simulink model "SimplerFFTV2"  (R2021b)
settings: Solver=VariableStepAuto  StartTime=0.0  StopTime=3*900/fs  RelTol=1e-3
InitFcn:
  | f = 1000;
  | fs = 18*f;
  | N = 10*fs/f;
  | n = 0:N-1;
  | Ts = 1/fs;
  | t = n*Ts
  | y_n = sin(2*pi*f*n*Ts);
  | Hann = 0.5 * (1 - cos(2*pi*(n/N)))
  | Hamming = 0.54 - 0.46*cos(2*pi*n/N)
undefined symbols (not defined in the file): y_n_Hamming_1Period
libraries: hdlBasic x12, vmcUtilities x1
settings Model: Creator=yxb20126  LastModifiedBy=yxb20126

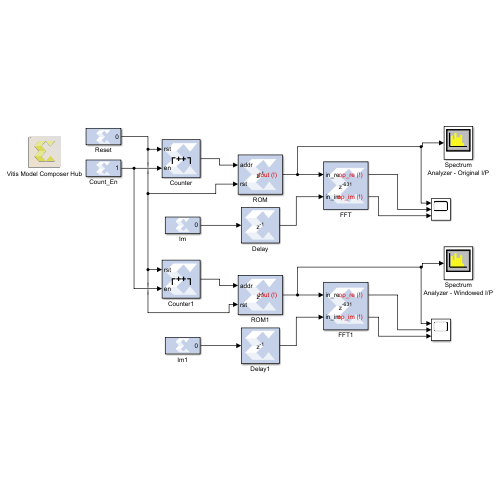
[thumbnail: Simulink's stored preview of the top-level diagram]
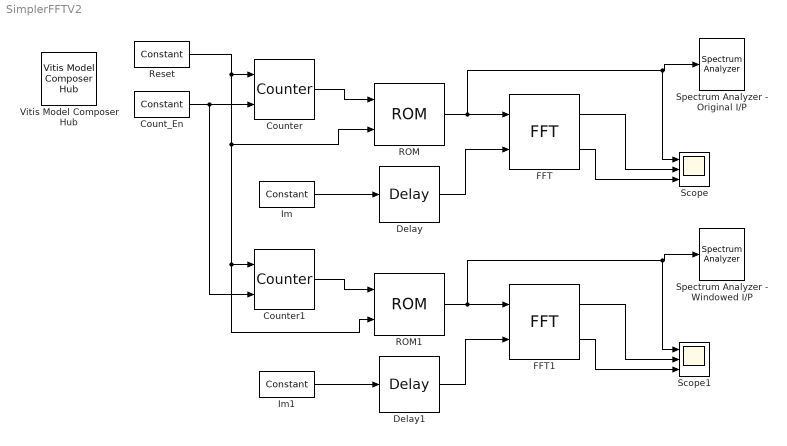
== system SimplerFFTV2 ==
  Count_En : hdlBasic/Constant  const=1  gui_display_data_type=Boolean  arith_type=Boolean  n_bits=16  bin_pt=14  preci_type=Single  exp_width=8  frac_width=24  explicit_period=on  period=1/fs  XmcBlockStatus=1  maskContainerNames=tabcontainer1  block_type=constant  block_config=sysgen:Constant_config
  Counter : hdlBasic/Counter  cnt_type=Count limited  cnt_to=length(y_n)-1  operation=Up  start_count=0  cnt_by_val=1  arith_type=Unsigned  n_bits=8  bin_pt=0  load_pin=off  rst=on  en=on  explicit_period=Explicit  period=1/fs  use_behavioral_HDL=off  implementation=Fabric  XmcBlockStatus=1  maskContainerNames=group1  block_type=counter  block_config=sysgen:Counter_config
  Counter1 : hdlBasic/Counter  cnt_type=Count limited  cnt_to=length(y_n_Hamming_1Period)-1  operation=Up  start_count=0  cnt_by_val=1  arith_type=Unsigned  n_bits=10  bin_pt=0  load_pin=off  rst=on  en=on  explicit_period=Explicit  period=1/fs  use_behavioral_HDL=off  implementation=Fabric  XmcBlockStatus=1  maskContainerNames=group1  block_type=counter  block_config=sysgen:Counter_config
  Delay : hdlBasic/Delay  rst=off  en=off  latency=1  reg_retiming=off  XmcBlockStatus=1  maskContainerNames=group1  block_type=delay  block_config=sysgen:Delay_config
  Delay1 : hdlBasic/Delay  rst=off  en=off  latency=1  reg_retiming=off  XmcBlockStatus=1  maskContainerNames=group1  block_type=delay  block_config=sysgen:Delay_config
  FFT : hdlBasic/FFT  transform_length=512  scale_result_by_fft_length=off  bit_reversed_order=off  optimizegoal=Performance  start_frame=off  simulation_type=fast_sim  simulation_model=sysgen:ForwardFFT_Macro  latency=1  XmcBlockStatus=1  maskContainerNames=group1  block_type=xfft_forward  block_config=sysgen:FFTMacro_config
  FFT1 : hdlBasic/FFT  transform_length=512  scale_result_by_fft_length=off  bit_reversed_order=off  optimizegoal=Performance  start_frame=off  simulation_type=fast_sim  simulation_model=sysgen:ForwardFFT_Macro  latency=1  XmcBlockStatus=1  maskContainerNames=group1  block_type=xfft_forward  block_config=sysgen:FFTMacro_config
  Im : hdlBasic/Constant  const=0  gui_display_data_type=Fixed-point  arith_type=Signed (2's comp)  n_bits=16  bin_pt=15  preci_type=Single  exp_width=8  frac_width=24  explicit_period=on  period=1/fs  XmcBlockStatus=1  maskContainerNames=tabcontainer1  block_type=constant  block_config=sysgen:Constant_config
  Im1 : hdlBasic/Constant  const=0  gui_display_data_type=Fixed-point  arith_type=Signed (2's comp)  n_bits=16  bin_pt=15  preci_type=Single  exp_width=8  frac_width=24  explicit_period=on  period=1/fs  XmcBlockStatus=1  maskContainerNames=tabcontainer1  block_type=constant  block_config=sysgen:Constant_config
  ROM : hdlBasic/ROM  depth=length(y_n)  initVector=y_n  distributed_mem=Block RAM  rst=on  init_reg=0  en=off  latency=1  gui_display_data_type=Fixed-point  arith_type="Signed  (2's comp)"  n_bits=16  bin_pt=15  preci_type=Double  exp_width=8  frac_width=24  optimize=Area  use_rpm=on  simulation_type=fast_sim  XmcBlockStatus=1  maskContainerNames=tabcontainer1  block_type=sprom  block_config=sysgen:SPROM_config
  ROM1 : hdlBasic/ROM  depth=length(y_n_Hamming_1Period)  initVector=y_n_Hamming_1Period  distributed_mem=Block RAM  rst=on  init_reg=0  en=off  latency=1  gui_display_data_type=Fixed-point  arith_type="Signed  (2's comp)"  n_bits=16  bin_pt=15  preci_type=Double  exp_width=8  frac_width=24  optimize=Area  use_rpm=on  simulation_type=fast_sim  XmcBlockStatus=1  maskContainerNames=tabcontainer1  block_type=sprom  block_config=sysgen:SPROM_config
  Reset : hdlBasic/Constant  const=0  gui_display_data_type=Boolean  arith_type=Boolean  n_bits=16  bin_pt=14  preci_type=Single  exp_width=8  frac_width=24  explicit_period=on  period=1/fs  XmcBlockStatus=1  maskContainerNames=tabcontainer1  block_type=constant  block_config=sysgen:Constant_config
  Scope : Scope  NumInputPorts=3
  Scope1 : Scope  NumInputPorts=3
  Spectrum Analyzer - Original I/P : SpectrumAnalyzer
  Spectrum Analyzer - Windowed I/P : SpectrumAnalyzer
  Vitis Model Composer Hub : vmcUtilities/Vitis Model Composer Hub  Tag=genX  CodeGeneration=off  SubsystemName=<enter or select subsystem name>  TargetDirectory=./code  ExportType=HLS C++ code  IpVendor=xilinx.com  IpLibrary=hls  IpVersion=1.0  IpHWLanguage=Verilog  AieCompilerOptions={}  CreateTestbench=off  TestbenchStackSize=10  RunAieSim=off  AieSimTimeout=50000  RunAieSimProfiling=off  LaunchVitisAnalyzer=off  PlotOutput=off  RunX86Sim=off  X86SimTimeout=10  GenHwImage=off  PlatformType=Not Specified  HwSystemType=Baremetal  HwValidationTarget=hw  ProjDevice=xczu48dr-fsvg1517-2-e  ProjDevicePart=xczu48dr-fsvg1517-2-e  SamplePeriod=-1  ClockFrequency=200  DataPathParallelism=1  xilinxfamily=zynquplusRFSOC  part=xczu48dr  speed=-2-e  package=fsvg1517  directory=./netlist  testbench=off  incr_netlist=off  synthesis_tool=Vivado  clock_wrapper=Clock Enables  dbl_ovrd=According to Block Masks  dcm_input_clock_period=10  sysclk_period=10  simulink_period=1/fs  eval_field=0
  wires:
  Delay/1 -> FFT/2
  Count_En/1 -> Counter1/2, Counter/2
  FFT/2 -> Scope/3
  FFT/1 -> Scope/2
  ROM/1 -> Spectrum Analyzer - Original I/P/1, Scope/1, FFT/1
  Counter/1 -> ROM/1
  Im/1 -> Delay/1
  Im1/1 -> Delay1/1
  Counter1/1 -> ROM1/1
  ROM1/1 -> FFT1/1, Scope1/1, Spectrum Analyzer - Windowed I/P/1
  FFT1/1 -> Scope1/2
  FFT1/2 -> Scope1/3
  Delay1/1 -> FFT1/2
  Reset/1 -> Counter/1, Counter1/1, ROM1/2, ROM/2
